simulink model "modelo_d"  (R2026a)
settings: Solver=VariableStepAuto  StopTime=60
values from neighbouring files (symbols this model uses):
  theta = 5    [init.m]
settings Model: Creator=honda  LastModifiedBy=honda

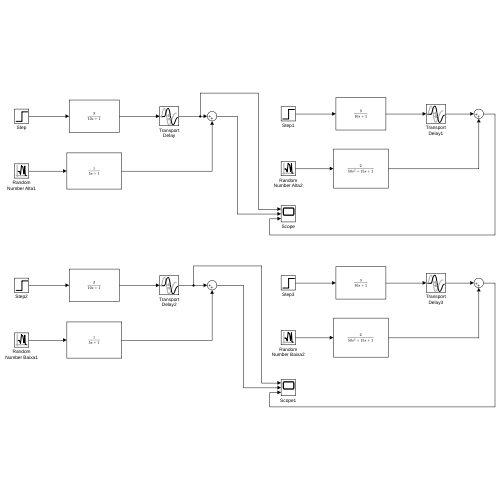
[thumbnail: Simulink's stored preview of the top-level diagram]
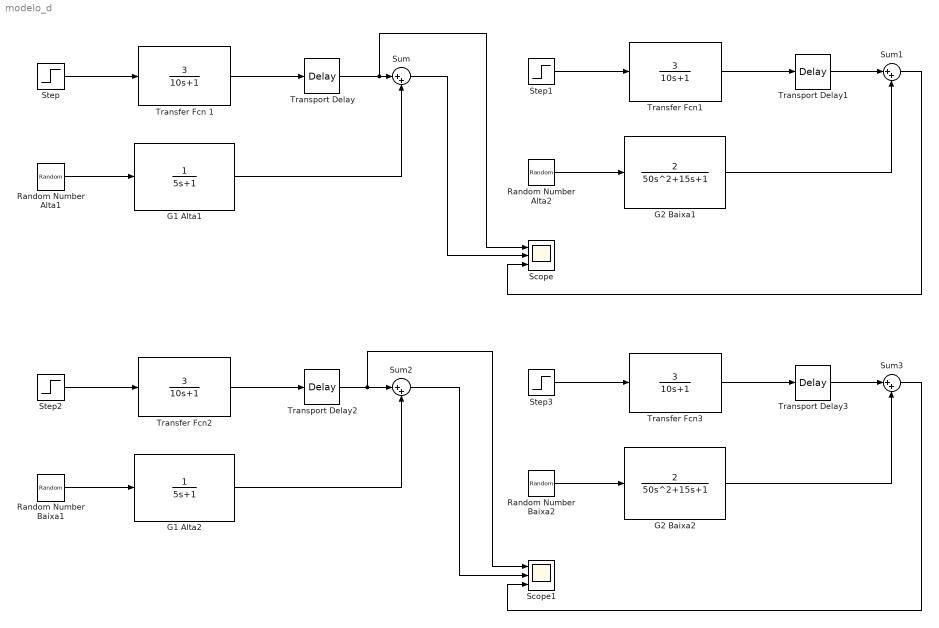
== system modelo_d ==
  G1 Alta1 : TransferFcn  Denominator=[5 1]
  G1 Alta2 : TransferFcn  Denominator=[5 1]
  G2 Baixa1 : TransferFcn  Numerator=[2]  Denominator=[50 15 1]
  G2 Baixa2 : TransferFcn  Numerator=[2]  Denominator=[50 15 1]
  Random Number Alta1 : RandomNumber  Variance=0.1  SampleTime=1
  Random Number Alta2 : RandomNumber  Variance=0.1  SampleTime=1
  Random Number Baixa1 : RandomNumber  Variance=0.001  SampleTime=1
  Random Number Baixa2 : RandomNumber  Variance=0.001  SampleTime=1
  Scope : Scope  NumInputPorts=3
      settings: ActiveDisplayYMinimum=-1  ActiveDisplayYMaximum=1  DataLoggingVariableName=dados_d_alta
  Scope1 : Scope  NumInputPorts=3
      settings: ActiveDisplayYMinimum=-1  ActiveDisplayYMaximum=1  DataLoggingVariableName=dados_d_baixa
  Step{,1..3} (4 alike) : Step  Time=0  FinalValue=u0  SampleTime=0
  Sum{,1..3} (4 alike) : Sum  Inputs=|++
  "Transfer Fcn 1 " : TransferFcn  Numerator=[3]  Denominator=[10 1]
  Transfer Fcn1 : TransferFcn  Numerator=[3]  Denominator=[10 1]
  Transfer Fcn2 : TransferFcn  Numerator=[3]  Denominator=[10 1]
  Transfer Fcn3 : TransferFcn  Numerator=[3]  Denominator=[10 1]
  Transport Delay{,1..3} (4 alike) : TransportDelay  DelayTime=theta
  wires:
  Transport Delay/1 -> Scope/1, Sum/1
  Step/1 -> "Transfer Fcn 1 "/1
  Sum/1 -> Scope/2
  "Transfer Fcn 1 "/1 -> Transport Delay/1
  Random Number Alta1/1 -> G1 Alta1/1
  G1 Alta1/1 -> Sum/2
  Step1/1 -> Transfer Fcn1/1
  Transport Delay1/1 -> Sum1/1
  Sum1/1 -> Scope/3
  Transfer Fcn1/1 -> Transport Delay1/1
  Random Number Alta2/1 -> G2 Baixa1/1
  G2 Baixa1/1 -> Sum1/2
  Step2/1 -> Transfer Fcn2/1
  Transport Delay2/1 -> Scope1/1, Sum2/1
  Sum2/1 -> Scope1/2
  Transfer Fcn2/1 -> Transport Delay2/1
  Random Number Baixa1/1 -> G1 Alta2/1
  G1 Alta2/1 -> Sum2/2
  Step3/1 -> Transfer Fcn3/1
  Random Number Baixa2/1 -> G2 Baixa2/1
  Transfer Fcn3/1 -> Transport Delay3/1
  Transport Delay3/1 -> Sum3/1
  Sum3/1 -> Scope1/3
  G2 Baixa2/1 -> Sum3/2
